simulink model "TFlex_basis"  (R2018b)
settings: Solver=VariableStepAuto  StartTime=0.0  StopTime=t_sim  RelTol=1e-3
values from neighbouring files (symbols this model uses):
  a0 = omega_n^3    (= 31006276.6803)    [initializeComparison.m]
  a1 = 3*omega_n^2    (= 296088.132033)    [initializeComparison.m]
  a2 = 3*omega_n    (= 942.477796077)    [initializeComparison.m]
  d_est = 0    [initializeComparison.m]
  f = xTrain(:,i_f)'    [TFlex_IFITC_compare.m]    (also in initializeComparison.m)
  h = 10*ts    (= 0.01)    [initializeComparison.m]
  I_limit = 2000    [initializeComparison.m]
  k_est = 0    [initializeComparison.m]
  Kd = kp*(tau_z-tau_p*(1+(tau_z+tau_p)/tau_i))    [initializeComparison.m]
  Ki = kp/tau_i    [initializeComparison.m]
  Kp = kp*(1+(tau_z-tau_p)/tau_i)    [initializeComparison.m]
  m_est = 0.2    [initializeComparison.m]
  p = [0, 0, -5, 0, 2]    [initializeComparison.m]
  r = 1e2    (= 100)    [initializeComparison.m]
  seed = 1    [initializeComparison.m]
  sp_ts = 1    [initializeComparison.m]
  tm = 0.1    [initializeComparison.m]
  ts = 1/1000    (= 0.001)    [initializeComparison.m]
undefined symbols (not defined in the file or in its folder): DiscIntNeverNeededParam, LPden, LPnum, P_estden, P_estnum, Pden, Pnum
libraries: simulink x5
settings Model: Creator=wout7  LastModifiedBy=wout7

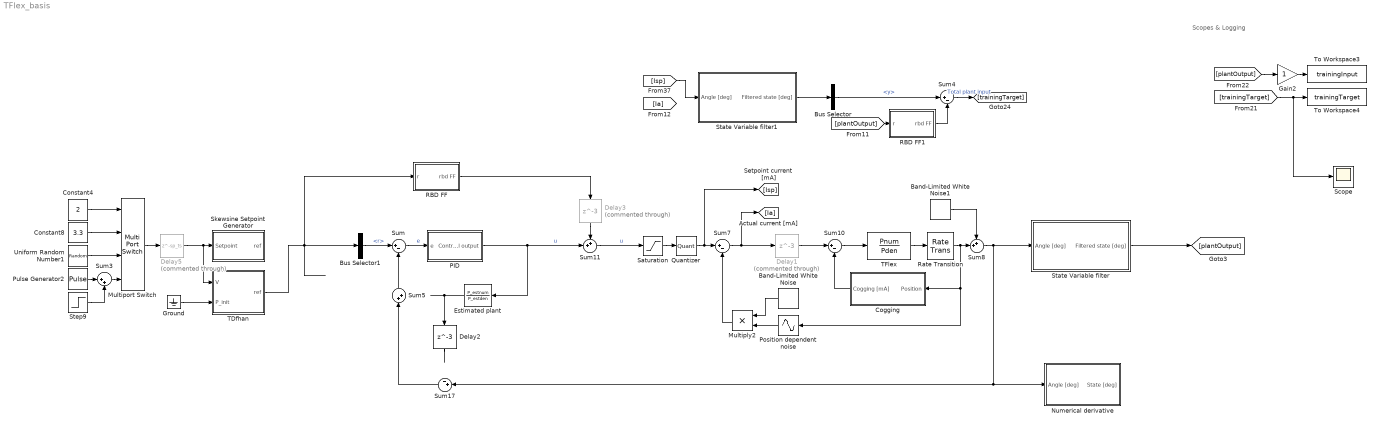
== system TFlex_basis ==
  note: Scopes & Logging
  Band-Limited White Noise : simulink/Sources/Band-Limited White Noise  Cov=[1e-3]  Ts=ts  seed=(seed+48124)
  Band-Limited White Noise1 : simulink/Sources/Band-Limited White Noise  Cov=[1e-15]  Ts=ts  seed=[23341]
  Bus Selector : BusSelector  OutputSignals=y
  Bus Selector1 : BusSelector  OutputSignals=r
  Cogging : Subsystem
  Constant4 : Constant  Value=2  SampleTime=sp_ts
  Constant8 : Constant  Value=3.3  SampleTime=sp_ts
  Delay1 : Delay  Commented=through  DelayLength=3  InitialCondition=0
  Delay2 : Delay  DelayLength=3  InitialCondition=0
  Delay3 : Delay  Commented=through  DelayLength=3  InitialCondition=0
  Delay5 : Delay  Commented=through  DelayLength=sp_ts  SampleTime=sp_ts
  Estimated plant : DiscreteTransferFcn  Numerator=P_estnum  Denominator=P_estden  SampleTime=ts
  Gain2 : Gain
  Ground : Ground
  Multiply2 : Product
  Multiport Switch : MultiPortSwitch
  Numerical derivative : Subsystem
  PID : Subsystem
  Position dependent noise : Sin  TimeSource=Use external signal  Amplitude=2.5  Bias=7.4979  Frequency=2*pi/13  SampleTime=0
  Pulse Generator2 : DiscretePulseGenerator  Amplitude=2*24  SampleTime=sp_ts
  Quantizer : Quantizer  QuantizationInterval=1
  RBD FF : Subsystem
  RBD FF1 : Subsystem
  Rate Transition : RateTransition  OutPortSampleTime=ts
  Saturation : Saturate  UpperLimit=I_limit  LowerLimit=-I_limit
  Scope : Scope
  Skewsine Setpoint Generator : Subsystem
  State Variable filter : Subsystem
  State Variable filter1 : Subsystem
  Step9 : Step  Time=0  After=-24  SampleTime=sp_ts
  Sum{,4,7,10} (4 alike) : Sum  Inputs=|+-
  Sum11 : Sum  Inputs=++|
  Sum17 : Sum  Inputs=-+|
  Sum3 : Sum  Inputs=|++
  Sum5 : Sum  Inputs=|++
  Sum8 : Sum  Inputs=++|
  TDfhan : Subsystem
  TFlex : TransferFcn  Numerator=Pnum  Denominator=Pden  ContinuousStateAttributes='angle'
  To Workspace3 : ToWorkspace  VariableName=trainingInput  SampleTime=-1
  To Workspace4 : ToWorkspace  VariableName=trainingTarget  SampleTime=-1
  Uniform Random Number1 : UniformRandomNumber  Minimum=-20  Maximum=20  Seed=seed  SampleTime=sp_ts
  wires:
  Sum/1 -> PID/1(e)  "e"
  Sum5/1 -> Sum/2
  Bus Selector1/1 -> Sum/1  "<r>"
  [plantOutput] -> RBD FF1/1(r)
  TFlex/1 -> Rate Transition/1
  [plantOutput] -> Gain2/1
  Gain2/1 -> To Workspace3/1
  TDfhan/1(ref) -> RBD FF/1(r), Bus Selector1/1
  Sum4/1 -> [trainingTarget]  "Total plant input"
  Saturation/1 -> Quantizer/1
  PID/1(Control output) -> Estimated plant/1, Sum11/2  "u"
  Estimated plant/1 -> Delay2/1
  Sum17/1 -> Sum5/1
  State Variable filter/1(Filtered state [deg]) -> [plantOutput]
  Rate Transition/1 -> Sum8/2, Cogging/1(Position), Position dependent noise/1
  Sum11/1 -> Saturation/1  "u"
  Sum8/1 -> Sum17/2, Numerical derivative/1(Angle [deg]), State Variable filter/1(Angle [deg])
  Sum10/1 -> TFlex/1
  Delay2/1 -> ?
  RBD FF1/1(rbd FF) -> Sum4/2
  State Variable filter1/1(Filtered state [deg]) -> Bus Selector/1
  Sum7/1 -> Delay1/1, [Ia]
  Multiply2/1 -> Sum7/2
  Cogging/1(Cogging [mA]) -> Sum10/2
  Quantizer/1 -> [Isp], Sum7/1
  RBD FF/1(rbd FF) -> Delay3/1
  Delay3/1 -> Sum11/1
  Band-Limited White Noise/1 -> Multiply2/1
  Position dependent noise/1 -> Multiply2/2
  Pulse Generator2/1 -> Sum3/1
  Sum3/1 -> Multiport Switch/4
  Step9/1 -> Sum3/2
  Constant4/1 -> Multiport Switch/1
  Uniform Random Number1/1 -> Multiport Switch/3
  Constant8/1 -> Multiport Switch/2
  Multiport Switch/1 -> Delay5/1
  Band-Limited White Noise1/1 -> Sum8/1
  Delay1/1 -> Sum10/1
  Delay5/1 -> TDfhan/1(V), Skewsine Setpoint Generator/1(Setpoint)
  [Isp] -> State Variable filter1/1(Angle [deg])
  Bus Selector/1 -> Sum4/1  "<y>"
  Ground/1 -> TDfhan/2(P_init)
  [trainingTarget] -> Scope/1, To Workspace4/1

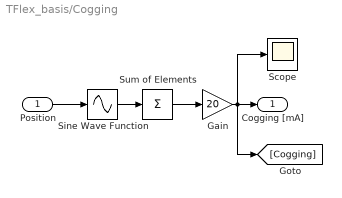
== system TFlex_basis/Cogging ==
  Position : Inport
  Gain : Gain  Gain=20
  Scope : Scope
  Sine Wave Function : Sin  TimeSource=Use external signal  Amplitude=a'  Frequency=2*pi./f'  Phase=p'*2*pi  SampleTime=0
  Sum of Elements : Sum  Inputs=+
  Cogging [mA] : Outport
  wires:
  Gain/1 -> Scope/1, [Cogging], Cogging [mA]/1
  Sum of Elements/1 -> Gain/1
  Position/1 -> Sine Wave Function/1
  Sine Wave Function/1 -> Sum of Elements/1

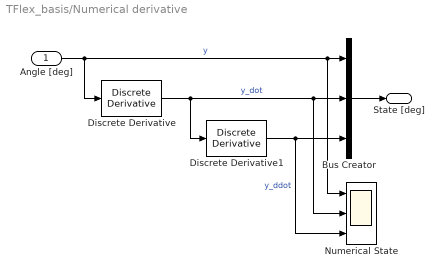
== system TFlex_basis/Numerical derivative ==
  Angle [deg] : Inport
  Bus Creator : BusCreator  Inputs=3
  Discrete Derivative : simulink/Discrete/Discrete Derivative  gainval=1.0  ICPrevScaledInput=0.0  OutMin=[]  OutMax=[]  OutDataType=fixdt(1, 16)  OutScaling=2^-10  DoSatur=off
  Discrete Derivative1 : simulink/Discrete/Discrete Derivative  gainval=1.0  ICPrevScaledInput=0.0  OutMin=[]  OutMax=[]  OutDataType=fixdt(1, 16)  OutScaling=2^-10  DoSatur=off
  Numerical State : Scope  NumInputPorts=3
  State [deg] : Outport
  wires:
  Discrete Derivative/1 -> Numerical State/2, Bus Creator/2, Discrete Derivative1/1  "y_dot"
  Angle [deg]/1 -> Numerical State/1, Bus Creator/1, Discrete Derivative/1  "y"
  Bus Creator/1 -> State [deg]/1
  Discrete Derivative1/1 -> Numerical State/3, Bus Creator/3  "y_ddot"

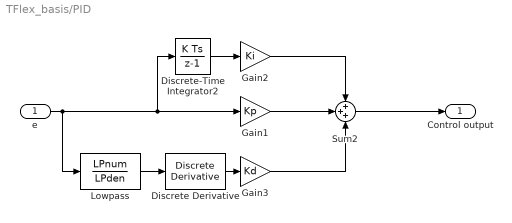
== system TFlex_basis/PID ==
  e : Inport
  Discrete Derivative : simulink/Discrete/Discrete Derivative  gainval=1.0  ICPrevScaledInput=0.0  OutMin=[]  OutMax=[]  OutDataType=fixdt(1, 16)  OutScaling=2^-10  DoSatur=off
  Discrete-Time Integrator2 : DiscreteIntegrator  SampleTime=-1  ICPrevOutput=DiscIntNeverNeededParam  ICPrevScaledInput=DiscIntNeverNeededParam
  Gain1 : Gain  Gain=Kp
  Gain2 : Gain  Gain=Ki
  Gain3 : Gain  Gain=Kd
  Lowpass : DiscreteTransferFcn  Numerator=LPnum  Denominator=LPden  SampleTime=ts
  Sum2 : Sum  Inputs=3
  Control output : Outport
  wires:
  Discrete-Time Integrator2/1 -> Gain2/1
  Gain1/1 -> Sum2/2
  Gain2/1 -> Sum2/1
  Gain3/1 -> Sum2/3
  Sum2/1 -> Control output/1
  e/1 -> Discrete-Time Integrator2/1, Gain1/1, Lowpass/1
  Lowpass/1 -> Discrete Derivative/1
  Discrete Derivative/1 -> Gain3/1

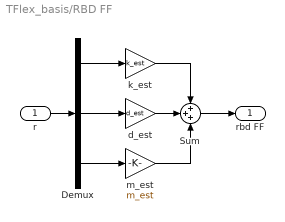
== system TFlex_basis/RBD FF ==
  r : Inport
  Demux : Demux  Outputs=3
  Sum : Sum  Inputs=+++
  d_est : Gain  Gain=d_est
  k_est : Gain  Gain=k_est
  m_est : Gain  Gain=m_est
  rbd FF : Outport
  wires:
  Demux/1 -> k_est/1
  Demux/2 -> d_est/1
  Demux/3 -> m_est/1
  m_est/1 -> Sum/3
  r/1 -> Demux/1
  d_est/1 -> Sum/2
  k_est/1 -> Sum/1
  Sum/1 -> rbd FF/1

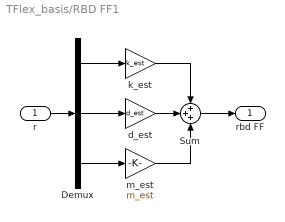
== system TFlex_basis/RBD FF1 ==
  r : Inport
  Demux : Demux  Outputs=3
  Sum : Sum  Inputs=+++
  d_est : Gain  Gain=d_est
  k_est : Gain  Gain=k_est
  m_est : Gain  Gain=m_est
  rbd FF : Outport
  wires:
  Demux/1 -> k_est/1
  Demux/2 -> d_est/1
  Demux/3 -> m_est/1
  m_est/1 -> Sum/3
  r/1 -> Demux/1
  d_est/1 -> Sum/2
  k_est/1 -> Sum/1
  Sum/1 -> rbd FF/1

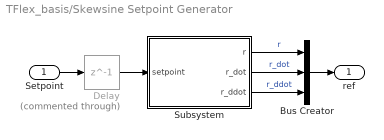
== system TFlex_basis/Skewsine Setpoint Generator ==
  Setpoint : Inport
  Bus Creator : BusCreator  Inputs=3
  Delay : Delay  Commented=through  DelayLength=1  InitialCondition=0
  Subsystem : Subsystem
  ref : Outport
  wires:
  Subsystem/3(r_ddot) -> Bus Creator/3  "r_ddot"
  Bus Creator/1 -> ref/1
  Setpoint/1 -> Delay/1
  Subsystem/2(r_dot) -> Bus Creator/2  "r_dot"
  Subsystem/1(r) -> Bus Creator/1  "r"
  Delay/1 -> Subsystem/1(setpoint)

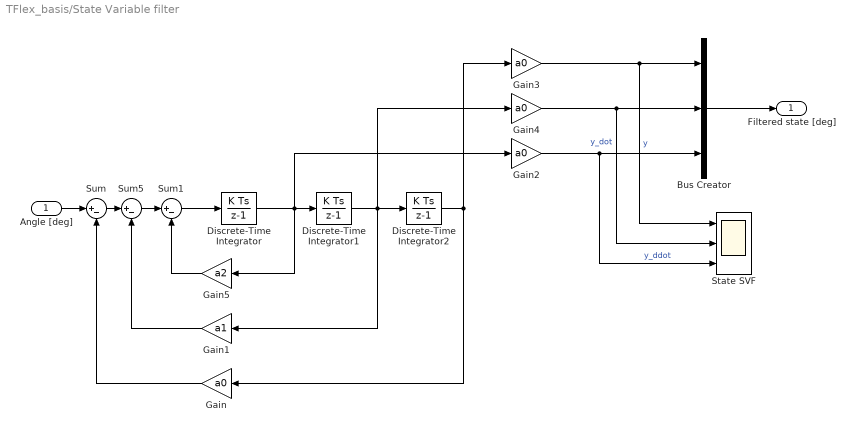
== system TFlex_basis/State Variable filter ==
  Angle [deg] : Inport
  Bus Creator : BusCreator  Inputs=3
  Discrete-Time Integrator : DiscreteIntegrator  SampleTime=-1  ICPrevOutput=DiscIntNeverNeededParam  ICPrevScaledInput=DiscIntNeverNeededParam
  Discrete-Time Integrator1 : DiscreteIntegrator  SampleTime=-1  ICPrevOutput=DiscIntNeverNeededParam  ICPrevScaledInput=DiscIntNeverNeededParam
  Discrete-Time Integrator2 : DiscreteIntegrator  SampleTime=-1  ICPrevOutput=DiscIntNeverNeededParam  ICPrevScaledInput=DiscIntNeverNeededParam
  Gain{,2..4} (4 alike) : Gain  Gain=a0
  Gain1 : Gain  Gain=a1
  Gain5 : Gain  Gain=a2
  State SVF : Scope  NumInputPorts=3
  Sum : Sum  Inputs=|+-
  Sum1 : Sum  Inputs=|+-
  Sum5 : Sum  Inputs=|+-
  Filtered state [deg] : Outport  SampleTime=ts
  wires:
  Bus Creator/1 -> Filtered state [deg]/1
  Sum1/1 -> Discrete-Time Integrator/1
  Angle [deg]/1 -> Sum/1
  Sum/1 -> Sum5/1
  Gain/1 -> Sum/2
  Gain1/1 -> Sum5/2
  Gain3/1 -> State SVF/1, Bus Creator/1  "y"
  Gain2/1 -> State SVF/3, Bus Creator/3  "y_ddot"
  Gain4/1 -> State SVF/2, Bus Creator/2  "y_dot"
  Gain5/1 -> Sum1/2
  Sum5/1 -> Sum1/1
  Discrete-Time Integrator/1 -> Discrete-Time Integrator1/1, Gain2/1, Gain5/1
  Discrete-Time Integrator1/1 -> Discrete-Time Integrator2/1, Gain4/1, Gain1/1
  Discrete-Time Integrator2/1 -> Gain3/1, Gain/1

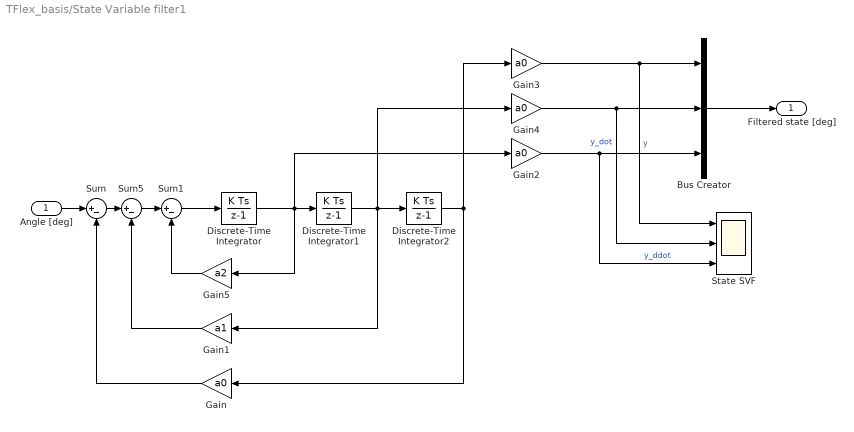
== system TFlex_basis/State Variable filter1 ==
  Angle [deg] : Inport
  Bus Creator : BusCreator  Inputs=3
  Discrete-Time Integrator : DiscreteIntegrator  SampleTime=-1  ICPrevOutput=DiscIntNeverNeededParam  ICPrevScaledInput=DiscIntNeverNeededParam
  Discrete-Time Integrator1 : DiscreteIntegrator  SampleTime=-1  ICPrevOutput=DiscIntNeverNeededParam  ICPrevScaledInput=DiscIntNeverNeededParam
  Discrete-Time Integrator2 : DiscreteIntegrator  SampleTime=-1  ICPrevOutput=DiscIntNeverNeededParam  ICPrevScaledInput=DiscIntNeverNeededParam
  Gain{,2..4} (4 alike) : Gain  Gain=a0
  Gain1 : Gain  Gain=a1
  Gain5 : Gain  Gain=a2
  State SVF : Scope  NumInputPorts=3
  Sum : Sum  Inputs=|+-
  Sum1 : Sum  Inputs=|+-
  Sum5 : Sum  Inputs=|+-
  Filtered state [deg] : Outport  SampleTime=ts
  wires:
  Bus Creator/1 -> Filtered state [deg]/1
  Sum1/1 -> Discrete-Time Integrator/1
  Angle [deg]/1 -> Sum/1
  Sum/1 -> Sum5/1
  Gain/1 -> Sum/2
  Gain1/1 -> Sum5/2
  Gain3/1 -> State SVF/1, Bus Creator/1  "y"
  Gain2/1 -> State SVF/3, Bus Creator/3  "y_ddot"
  Gain4/1 -> State SVF/2, Bus Creator/2  "y_dot"
  Gain5/1 -> Sum1/2
  Sum5/1 -> Sum1/1
  Discrete-Time Integrator/1 -> Discrete-Time Integrator1/1, Gain2/1, Gain5/1
  Discrete-Time Integrator1/1 -> Discrete-Time Integrator2/1, Gain4/1, Gain1/1
  Discrete-Time Integrator2/1 -> Gain3/1, Gain/1

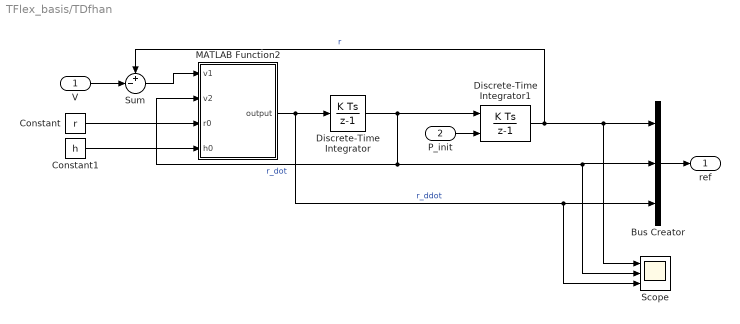
== system TFlex_basis/TDfhan ==
  V : Inport
  P_init : Inport  Port=2
  Bus Creator : BusCreator  Inputs=3
  Constant : Constant  Value=r  SampleTime=ts
  Constant1 : Constant  Value=h  SampleTime=ts
  Discrete-Time Integrator : DiscreteIntegrator  gainval=1  SampleTime=ts  ICPrevOutput=DiscIntNeverNeededParam  ICPrevScaledInput=DiscIntNeverNeededParam
  Discrete-Time Integrator1 : DiscreteIntegrator  gainval=1  InitialConditionSource=external  InitialCondition=-24  SampleTime=ts  ICPrevOutput=DiscIntNeverNeededParam  ICPrevScaledInput=DiscIntNeverNeededParam
  MATLAB Function2 : MATLAB Function  TreatAsAtomicUnit=on
  Scope : Scope  NumInputPorts=3
  Sum : Sum  Inputs=+-|
  ref : Outport
  wires:
  Sum/1 -> MATLAB Function2/1(v1)
  V/1 -> Sum/2
  Constant/1 -> MATLAB Function2/3(r0)
  Constant1/1 -> MATLAB Function2/4(h0)
  P_init/1 -> Discrete-Time Integrator1/2
  Discrete-Time Integrator1/1 -> Sum/1, Scope/1, Bus Creator/1  "r"
  Discrete-Time Integrator/1 -> Discrete-Time Integrator1/1, Scope/2, Bus Creator/2, MATLAB Function2/2(v2)  "r_dot"
  Bus Creator/1 -> ref/1
  MATLAB Function2/1(output) -> Scope/3, Bus Creator/3, Discrete-Time Integrator/1  "r_ddot"

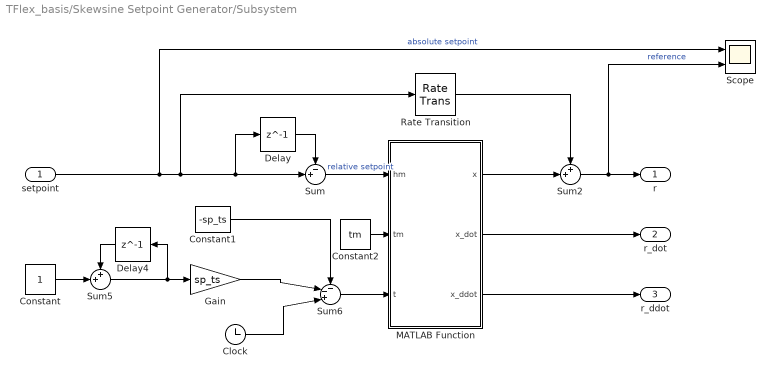
== system TFlex_basis/Skewsine Setpoint Generator/Subsystem ==
  setpoint : Inport
  Clock : Clock
      settings: Decimation=100
  Constant : Constant  SampleTime=sp_ts
  Constant1 : Constant  Value=-sp_ts  SampleTime=sp_ts
  Constant2 : Constant  Value=tm  SampleTime=sp_ts
  Delay : Delay  DelayLength=1  InitialCondition=0  SampleTime=sp_ts
  Delay4 : Delay  DelayLength=1  InitialCondition=0  SampleTime=sp_ts
  Gain : Gain  Gain=sp_ts
  MATLAB Function : MATLAB Function  TreatAsAtomicUnit=on
  Rate Transition : RateTransition  OutPortSampleTime=ts
  Scope : Scope  NumInputPorts=2
  Sum : Sum  Inputs=-+|
  Sum2 : Sum  Inputs=++|
  Sum5 : Sum  Inputs=++|
  Sum6 : Sum  Inputs=--+|
  r : Outport
  r_dot : Outport  Port=2
  r_ddot : Outport  Port=3
  wires:
  Delay4/1 -> Sum5/1
  Sum2/1 -> r/1, Scope/2  "reference"
  Sum5/1 -> Delay4/1, Gain/1
  Constant/1 -> Sum5/2
  MATLAB Function/3(x_ddot) -> r_ddot/1
  Clock/1 -> Sum6/3
  Delay/1 -> Sum/1
  Gain/1 -> Sum6/2
  Constant1/1 -> Sum6/1
  MATLAB Function/2(x_dot) -> r_dot/1
  Sum/1 -> MATLAB Function/1(hm)  "relative setpoint"
  Constant2/1 -> MATLAB Function/2(tm)
  Sum6/1 -> MATLAB Function/3(t)
  MATLAB Function/1(x) -> Sum2/2
  setpoint/1 -> Scope/1, Rate Transition/1, Delay/1, Sum/2  "absolute setpoint"
  Rate Transition/1 -> Sum2/1

== matlab function TFlex_basis/Skewsine Setpoint Generator/Subsystem/MATLAB Function ==
  settings: updateMethod=DISCRETE  sampleTime=ts
  data: hm input; x output; tm input; t input; x_dot output; x_ddot output
function [x,x_dot,x_ddot] = skewSine(hm,tm,t)

if (t>=0) && (t<=tm)
    x      = hm/tm*t - hm/(2*pi)*sin(2*pi/tm*t);
    x_dot  = hm/tm - hm/tm*cos(2*pi/tm*t);
    x_ddot = 2*pi*hm/(tm^2)*sin(2*pi/tm*t);
else
    x      = hm;
    x_dot  = 0;
    x_ddot = 0;
end

== matlab function TFlex_basis/TDfhan/MATLAB Function2 ==
  data: v1 input; output output; v2 input; r0 input; h0 input
function output = Fhan(v1,v2,r0, h0)
d = h0^2*r0;
a0 = h0*v2;
y = v1 + a0;
a1 = sqrt(d*(d+8*abs(y)));
a2 = a0 + sign(y)*(a1-d)/2;
sy = (sign(y+d)-sign(y-d))/2;
a = (a0+y-a2)*sy +a2;
sa = (sign(a+d)-sign(a-d))/2;
output = -r0 *(a/d -sign(a) )*sa - r0*sign(a);
